simulink model "TransferenciaP2"  (Simulink 9.1)
settings: Solver=VariableStepAuto  StartTime=0.0  StopTime=10.0  RelTol=1e-3
values from neighbouring files (symbols this model uses):
  kp = 1000    [Problema2TF.m]    (also in Problema2itemi.m)
settings Model: Creator=valen  LastModifiedBy=valen
settings DataIOCC: SaveFormat=Dataset
settings OptimizationCC: LifeSpan=auto
settings DebuggingCC: UnderspecifiedInitializationDetection=Simplified  MergeDetectMultiDrivingBlocksExec=error  SFUnexpectedBacktrackingDiag=error  SFNoUnconditionalDefaultTransitionDiag=error  SFExecutionAtInitializationDiag=warning
settings HardwareCC: ProdBitPerPointer=64  ProdBitPerSizeT=64  ProdBitPerPtrDiffT=64  ProdLargestAtomicFloat=Float  ProdIntDivRoundTo=Zero  ProdEndianess=LittleEndian  ProdWordSize=64  ProdHWDeviceType=Intel->x86-64 (Windows64)
settings ModelReferenceCC: PropagateSignalLabelsOutOfModel=on
settings CodeAppCC: StateflowObjectComments=off
settings GRTTargetCC: TargetLangStandard=C99 (ISO)  CombineOutputUpdateFcns=on  GRTInterface=off
settings ConfigComp: CovMetricSettings=dwe  CovHtmlReporting=off  CovSaveCumulativeToWorkspaceVar=off  CovSaveSingleToWorkspaceVar=off  CovExternalEMLEnable=on

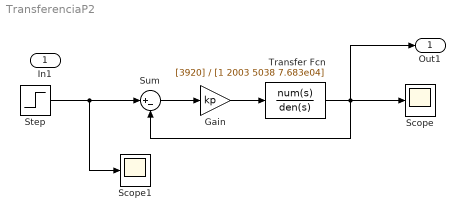
== system TransferenciaP2 ==
  In1 : Inport
  Gain : Gain  Gain=kp
  Scope : Scope
  Scope1 : Scope
  Step : Step  Time=0  Before=0.2  After=0.2  SampleTime=0
  Sum : Sum  Inputs=|+-
  Transfer Fcn : TransferFcn  Numerator=[3920]  Denominator=[1 2003 5038 7.683e04]
  Out1 : Outport
  wires:
  Transfer Fcn/1 -> Scope/1, Sum/2, Out1/1
  Sum/1 -> Gain/1
  Gain/1 -> Transfer Fcn/1
  Step/1 -> Scope1/1, Sum/1
